simulink model "QuadrotorExponentialTrackingController"  (R2021a)
settings: Solver=VariableStepAuto  StartTime=0.0  StopTime=100  MaxStep=0.001  MinStep=0.00011  RelTol=1e-2
undefined symbols (not defined in the file): DiscIntNeverNeededParam
libraries: simulink x3
settings Model: Creator=aruna  LastModifiedBy=aruna
settings SolverCC: MaxConsecutiveMinStep=5  ZeroCrossAlgorithm=Adaptive
settings DebuggingCC: ReadBeforeWriteMsg=DisableAll  WriteAfterWriteMsg=DisableAll  WriteAfterReadMsg=DisableAll  AlgebraicLoopMsg=none  ArtificialAlgebraicLoopMsg=none  MultiTaskDSMMsg=none
settings ModelReferenceCC: UpdateModelReferenceTargets=IfOutOfDate
settings SFSimCC: SFSimEcho=off

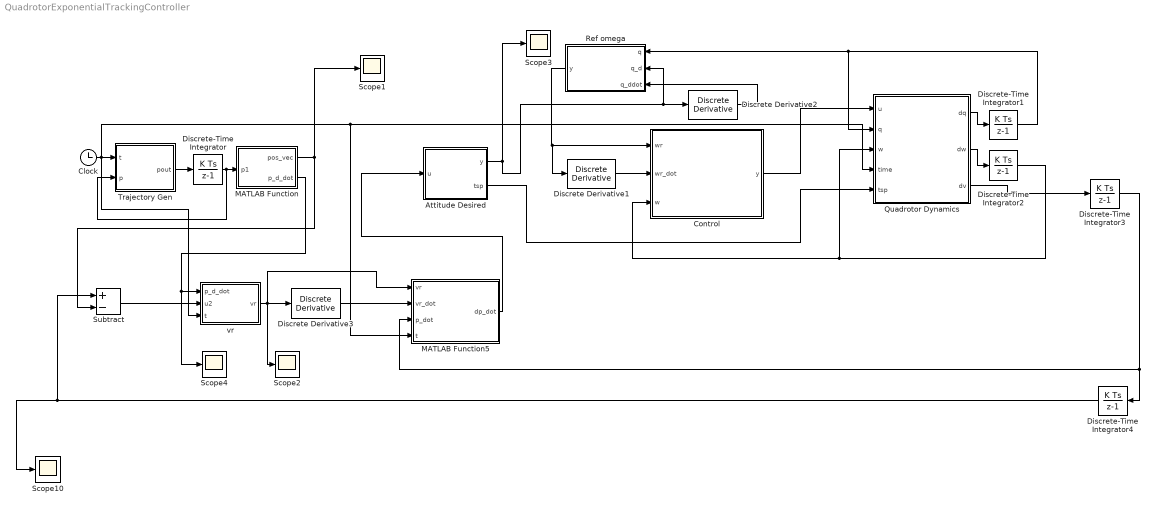
== system QuadrotorExponentialTrackingController ==
  Attitude Desired : MATLAB Function  TreatAsAtomicUnit=on
  Clock : Clock
  Control : MATLAB Function  TreatAsAtomicUnit=on
  Discrete Derivative1 : simulink/Discrete/Discrete Derivative  gainval=1.0  ICPrevScaledInput=0.0  OutMin=[]  OutMax=[]  OutDataType=fixdt(1, 16)  OutScaling=2^-10  DoSatur=off
  Discrete Derivative2 : simulink/Discrete/Discrete Derivative  gainval=1.0  ICPrevScaledInput=0.0  OutMin=[]  OutMax=[]  OutDataType=fixdt(1, 16)  OutScaling=2^-10  DoSatur=off
  Discrete Derivative3 : simulink/Discrete/Discrete Derivative  gainval=1.0  ICPrevScaledInput=0.0  OutMin=[]  OutMax=[]  OutDataType=fixdt(1, 16)  OutScaling=2^-10  DoSatur=off
  Discrete-Time Integrator{,1..4} (5 alike) : DiscreteIntegrator  SampleTime=-1  ICPrevOutput=DiscIntNeverNeededParam  ICPrevScaledInput=DiscIntNeverNeededParam
  MATLAB Function : MATLAB Function  TreatAsAtomicUnit=on
  MATLAB Function5 : MATLAB Function  TreatAsAtomicUnit=on
  Quadrotor Dynamics : MATLAB Function  TreatAsAtomicUnit=on
  Ref omega : MATLAB Function  TreatAsAtomicUnit=on
  Scope{1..4,10} (5 alike) : Scope
  Subtract : Sum  Inputs=+-
  Trajectory Gen : MATLAB Function  TreatAsAtomicUnit=on
  vr : MATLAB Function  TreatAsAtomicUnit=on
  wires:
  Ref omega/1(y) -> Discrete Derivative1/1, Control/1(wr)
  Trajectory Gen/1(pout) -> Discrete-Time Integrator/1
  Discrete Derivative1/1 -> Control/2(wr_dot)
  Discrete-Time Integrator2/1 -> Quadrotor Dynamics/3(w), Control/3(w)
  Clock/1 -> vr/3(t), Trajectory Gen/1(t), Quadrotor Dynamics/4(time), MATLAB Function5/4(t)
  Control/1(y) -> Quadrotor Dynamics/1(u)
  Discrete-Time Integrator1/1 -> Quadrotor Dynamics/2(q), Ref omega/1(q)
  MATLAB Function/1(pos_vec) -> Subtract/2, Scope1/1
  Attitude Desired/1(y) -> Discrete Derivative2/1, Ref omega/2(q_d), Scope3/1
  MATLAB Function/2(p_d_dot) -> Scope4/1, vr/1(p_d_dot)
  Discrete-Time Integrator/1 -> Trajectory Gen/2(p), MATLAB Function/1(p1)
  Quadrotor Dynamics/1(dq) -> Discrete-Time Integrator1/1
  MATLAB Function5/1(dp_dot) -> Attitude Desired/1(u)
  Discrete Derivative2/1 -> Ref omega/3(q_ddot)
  Quadrotor Dynamics/2(dw) -> Discrete-Time Integrator2/1
  Subtract/1 -> vr/2(u2)
  vr/1(vr) -> MATLAB Function5/1(vr), Discrete Derivative3/1, Scope2/1
  Discrete Derivative3/1 -> MATLAB Function5/2(vr_dot)
  Discrete-Time Integrator4/1 -> Scope10/1, Subtract/1
  Attitude Desired/2(tsp) -> Quadrotor Dynamics/5(tsp)
  Quadrotor Dynamics/3(dv) -> Discrete-Time Integrator3/1
  Discrete-Time Integrator3/1 -> MATLAB Function5/3(p_dot), Discrete-Time Integrator4/1

== matlab function QuadrotorExponentialTrackingController/Trajectory Gen ==
  data: t input; pout output; p input
function pout = fcn(t,p)
dt = 0.01;
time = t;
if time < 0.1
    present_state = [0;0;0;0;0;0];
end
present_state = p;
%p1 vector contains the position and velocity
x_present = [present_state(1);present_state(2)];
y_present = [present_state(3);present_state(4)];
z_present = [present_state(5);present_state(6)];

dx = x_pos(time,x_present);
dy = y_pos(time,y_present);
dz = z_pos(time,z_present);
pout = vertcat(dx,dy,dz);
end

function yout = rk4singlestep(fun,dt,tk,yk) 
f1 = fun(tk,yk);
f2 = fun(tk+dt/2,yk+(dt/2)*f1);
f3 = fun(tk+dt/2,yk+(dt/2)*f2);
f4 = fun(tk+dt,yk+dt*f3);

yout = yk + (dt/6)*(f1+2*f2+2*f3+f4);
end

function dx = x_pos(time,x)

dx = [x(2);4 - 3*x(2) - 2*x(1)];
end

function dy = y_pos(time,y)

dy = [y(2); 2 - 3*y(2) - 2*y(1)];
end

function dz = z_pos(time,z)

dz = [z(2);2 - 3*z(2) - 2*z(1)];
end

== matlab function QuadrotorExponentialTrackingController/Attitude Desired ==
  data: u input size=[3,1]; y output; tsp output
function [y,tsp]  = fcn(u)


X_bar = u(1);
Y_bar = u(2);
Z_bar = u(3) + 9.81;

Fd = sqrt((X_bar)^2 + (Y_bar)^2 + (Z_bar)^2 );

psi_d = 0;
phi_d = asin(-(Y_bar)/Fd);
theta_d = atan2((X_bar)/Z_bar,1);

q_d = [theta_d;phi_d;psi_d];
y = q_d ;
tsp = [0;0;Fd];

== matlab function QuadrotorExponentialTrackingController/Control ==
  data: wr input size=[3,1]; y output; wr_dot input size=[3,1]; w input size=[3,1]
function y = fcn(wr, wr_dot, w)
J = [1 0 0; 0 1 0; 0 0 1];
K = 4.4.*[1 0 0; 0 1 0; 0 0 1];



cross = J*w;
cross_skew = [0 -cross(3) cross(2);cross(3) 0 -cross(1);-cross(2) cross(1) 0];
u = J*wr_dot - cross_skew*wr - K*(w - wr);

y = u;

== matlab function QuadrotorExponentialTrackingController/Quadrotor Dynamics ==
  data: u input; q input size=[3,1]; w input size=[3,1]; dq output; dw output; time input; tsp input; dv output
function [dq,dw,dv] = fcn(u, q, w, time, tsp)
dt = 0.01;
if time < 0.01
    w = [0;0;0];
    q = [0;0;0];
end

dw = omega(w,u);
dq = attitude(q,w);
theta = q(1);
phi = q(2);
psi = q(3);
Z_q = [1 sin(phi)*tan(theta) cos(phi)*tan(theta);0 cos(phi) -sin(phi);0 sin(phi)*sec(theta) cos(phi)*sec(theta)];
dv = [0;0;-9.81] + (Z_q)*tsp;

end

function dw = omega(w,u)
J = [1 0 0;0 1 0;0 0 1];
omega = [w(1);w(2);w(3)];
cross = J*omega;
cross_skew = [0 -cross(3) cross(2);cross(3) 0 -cross(1);-cross(2) cross(1) 0];
dw = cross_skew*omega + u;
end

function dq = attitude(q,w)

theta = q(1);
phi = q(2);
psi = q(3);

Z_q = [1 sin(phi)*tan(theta) cos(phi)*tan(theta);0 cos(phi) -sin(phi);0 sin(phi)*sec(theta) cos(phi)*sec(theta)];
omega = [w(1);w(2);w(3)];
dq = Z_q*omega;
end

function yout = rk4singlestepat(fun,dt,yk,u) 
yk = [yk(1);yk(2);yk(3)];
f1 = fun(yk,u);
f2 = fun(yk+(dt/2)*f1,u);
f3 = fun(yk+(dt/2)*f2,u);
f4 = fun(yk+dt*f3,u);

yout = yk + (dt/6)*(f1+2*f2+2*f3+f4);
end

== matlab function QuadrotorExponentialTrackingController/Ref omega ==
  data: q input size=[3,1]; y output; q_d input; q_ddot input
function y = fcn(q, q_d, q_ddot)
theta = q(1);
phi = q(2);
psi = q(3);
att = [theta;phi;psi];
L = [1 0 0;0 1 0;0 0 1];%lambda parameter
J = [1 0 0;0 1 0;0 0 1];%inertia tensor

Z_q = [1 sin(phi)*tan(theta) cos(phi)*tan(theta);0 cos(phi) -sin(phi);0 sin(phi)*sec(theta) cos(phi)*sec(theta)];
w_r = Z_q\q_ddot + Z_q\L*(q_d - att);

y = w_r;

== matlab function QuadrotorExponentialTrackingController/MATLAB Function ==
  data: p1 input; pos_vec output; p_d_dot output
function [pos_vec,p_d_dot] = fcn(p1)
pos_vec = [p1(1);p1(3);p1(5)];
p_d_dot = [p1(2);p1(4);p1(6)];

== matlab function QuadrotorExponentialTrackingController/vr ==
  data: p_d_dot input; vr output size=[3,1]; u2 input; t input
function vr = fcn(p_d_dot,u2,t)
lambda = 1;

vr = p_d_dot - lambda*(u2);

== matlab function QuadrotorExponentialTrackingController/MATLAB Function5 ==
  data: vr input; dp_dot output size=[3,1]; vr_dot input; p_dot input; t input
function dp_dot = fcn(vr,vr_dot,p_dot,t)
if t < 0.1
    dp_dot = [0;0;0];
end
Kv = 1;
if t < 150
temp = -Kv*(p_dot - vr) + vr_dot;
dp_dot = temp;
else
dp_dot = [0;0;0];
end
